simulink model "trajectoryGenerator"  (R2021b)
settings: Solver=VariableStepAuto  StartTime=0.0  StopTime=10  RelTol=1e-3
settings Model: Creator=marcus  LastModifiedBy=marcus
settings OptimizationCC: BlockReduction=off  DefaultParameterBehavior=Inlined  BufferReuse=off

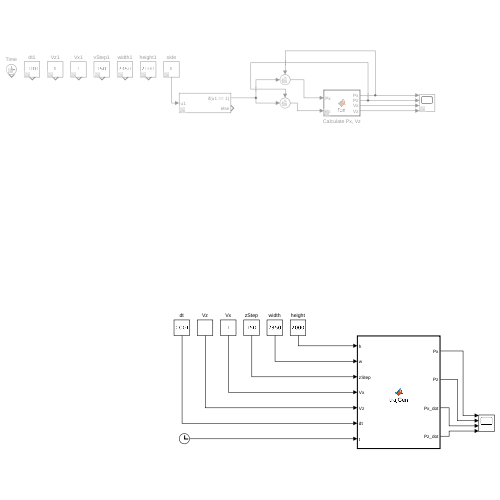
[thumbnail: Simulink's stored preview of the top-level diagram]
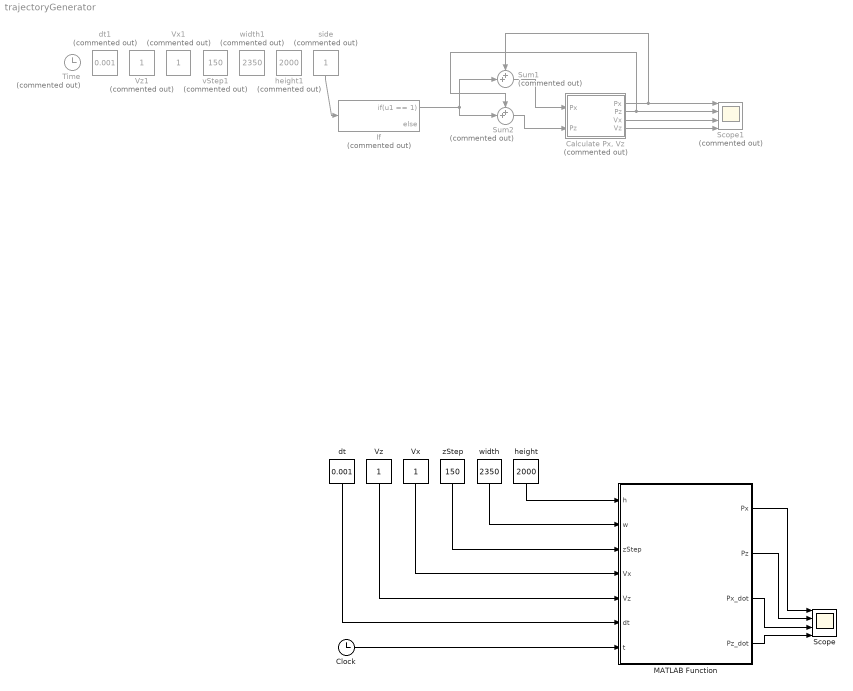
== system trajectoryGenerator ==
  "Calculate Px, Vz" : MATLAB Function  Commented=on  TreatAsAtomicUnit=on
  Clock : Clock
      settings: Decimation=2
  If : If  Commented=on  IfExpression=u1 == 1
  MATLAB Function : MATLAB Function  TreatAsAtomicUnit=on
  Scope : Scope  NumInputPorts=4
  Scope1 : Scope  Commented=on  NumInputPorts=4
  Sum1 : Sum  Commented=on  Inputs=++|
  Sum2 : Sum  Commented=on  Inputs=++|
  Time : Clock  Commented=on
  Vx : Constant
  Vx1 : Constant  Commented=on
  Vz : Constant
  Vz1 : Constant  Commented=on
  dt : Constant  Value=0.001
  dt1 : Constant  Commented=on  Value=0.001
  height : Constant  Value=2000
  height1 : Constant  Commented=on  Value=2000
  side : Constant  Commented=on
  vStep1 : Constant  Commented=on  Value=150
  width : Constant  Value=2350
  width1 : Constant  Commented=on  Value=2350
  zStep : Constant  Value=150
  wires:
  height/1 -> MATLAB Function/1(h)
  width/1 -> MATLAB Function/2(w)
  zStep/1 -> MATLAB Function/3(zStep)
  dt/1 -> MATLAB Function/6(dt)
  Vx/1 -> MATLAB Function/4(Vx)
  Vz/1 -> MATLAB Function/5(Vz)
  MATLAB Function/1(Px) -> Scope/1
  MATLAB Function/2(Pz) -> Scope/2
  MATLAB Function/3(Px_dot) -> Scope/3
  Clock/1 -> MATLAB Function/7(t)
  MATLAB Function/4(Pz_dot) -> Scope/4
  side/1 -> If/1
  "Calculate Px, Vz"/1(Px) -> Sum1/1, Scope1/1
  "Calculate Px, Vz"/4(Vz) -> Scope1/4
  "Calculate Px, Vz"/2(Pz) -> Sum2/1, Scope1/2
  If/1 -> Sum1/2, Sum2/2
  Sum2/1 -> "Calculate Px, Vz"/2("Pz ")
  Sum1/1 -> "Calculate Px, Vz"/1("Px ")
  "Calculate Px, Vz"/3(Vx) -> Scope1/3

== matlab function trajectoryGenerator/Calculate Px, Vz ==
  data: Px input; Px output; Pz output; Vx output; Pz input; Vz output
function [Px, Pz, Vx, Vz]= fcn(Px, Pz)

Px = Px + 1
Pz = Pz + 1
Vx = 1
Vz =1

== matlab function trajectoryGenerator/MATLAB Function ==
  data: h input; w input; zStep input; Vx input; Vz input; dt input; t input; Px output; Pz output; Px_dot output; Pz_dot output
function [Px, Pz, Px_dot, Pz_dot] = trajGen(h, w, zStep, Vx, Vz, dt, t)

Px = 0
if(t <= 2)
Px = tanh(t)
elseif(t >= 2 && t <= 6)
Px = tanh(t)
elseif(t >= 6 && t < 10)
Px = tanh(t)
end



Pz=0;
Px_dot=0;
Pz_dot=0;
end
